simulink model "Subsystem"  (R2020a)
settings: Solver=FixedStepAuto  StartTime=0.0  StopTime=10.0  FixedStep=0.001  RelTol=1e-3
settings Model: Creator=tnradm  LastModifiedBy=tnradm
settings DataIOCC: SaveOutput=off  SaveTime=off

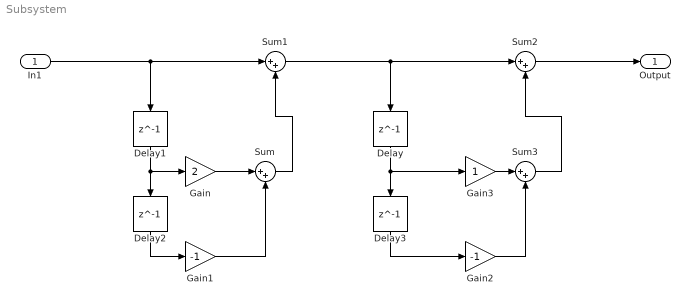
== system Subsystem ==
  In1 : Inport  OutDataTypeStr=double  PortDimensions=1  SampleTime=[0.001,0]
  Delay{,1..3} (4 alike) : Delay  DelayLength=1
  Gain : Gain  Gain=2
  Gain1 : Gain  Gain=-1
  Gain2 : Gain  Gain=-1
  Gain3 : Gain
  Sum{,1..3} (4 alike) : Sum  Inputs=|++
  Output : Outport  OutDataTypeStr=double  PortDimensions=1  SampleTime=[0.001,0]
  wires:
  Sum3/1 -> Sum2/2
  Sum/1 -> Sum1/2
  Delay/1 -> Gain3/1, Delay3/1
  Delay2/1 -> Gain1/1
  Gain3/1 -> Sum3/1
  Sum1/1 -> Sum2/1, Delay/1
  In1/1 -> Sum1/1, Delay1/1
  Delay1/1 -> Gain/1, Delay2/1
  Gain/1 -> Sum/1
  Gain1/1 -> Sum/2
  Gain2/1 -> Sum3/2
  Delay3/1 -> Gain2/1
  Sum2/1 -> Output/1
